simulink library "MotionSimSpatialLibrary"  (Simulink 7.8)
settings: Solver=ode45  StartTime=0.0  StopTime=10.0  RelTol=1e-3
values from neighbouring files (symbols this model uses):
  sysmodel = CalcDof( sysmodel)    [conv2simulink.m]
undefined symbols (not defined in the file or in its folder): selectnum
settings Model: Creator=john  LastModifiedBy=john

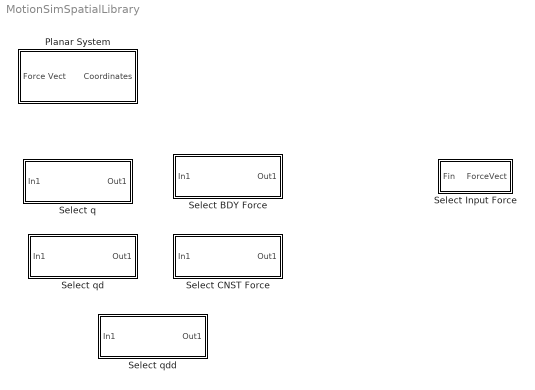
== system MotionSimSpatialLibrary ==
  Planar System : Subsystem
  Select BDY Force : Subsystem  mask{Bodynum=3, Selectnum=Tx}
      mask prompts: Bodynum "Body Number"; Selectnum "Select Coordinate"
      mask StyleString: edit,popup(Fx|Fy|Fz|Tx|Ty|Tz)
      mask Display:
      | port_label('input',1,'Coord');
      | port_label('output',1,'BDY Force');
  Select CNST Force : Subsystem  mask{Bodynum=1, Selectnum=Tx}
      mask prompts: Bodynum "Body Number"; Selectnum "Select Coordinate"
      mask StyleString: edit,popup(Fx|Fy|Fz|Tx|Ty|Tz)
      mask Display:
      | port_label('input',1,'Coord');
      | port_label('output',1,'CNST Force');
  Select Input Force : Subsystem  mask{BodyNum=1, ForceNum=Tx}
      mask prompts: BodyNum "Body Number"; ForceNum "Force"
      mask StyleString: edit,popup(Fx|Fy|Fz|Tx|Ty|Tz)
  Select q : Subsystem  mask{Bodynum=3, Selectnum=X}
      mask prompts: Bodynum "Body Number"; Selectnum "Select Coordinate"
      mask StyleString: edit,popup(X|Y|Z|e0|e1|e2|e3)
      mask Display:
      | port_label('input',1,'Coord');
      | port_label('output',1,'q');
  Select qd : Subsystem  mask{Bodynum=3, Selectnum=Xd}
      mask prompts: Bodynum "Body Number"; Selectnum "Select Coordinate"
      mask StyleString: edit,popup(Xd|Yd|Zd|e0d|e1d|e2d|e3d)
      mask Display:
      | port_label('input',1,'Coord');
      | port_label('output',1,'qd');
  Select qdd : Subsystem  mask{Bodynum=3, Selectnum=Xdd}
      mask prompts: Bodynum "Body Number"; Selectnum "Select Coordinate"
      mask StyleString: edit,popup(Xdd|Ydd|Zdd|e0dd|e1dd|e2dd|e3dd)
      mask Display:
      | port_label('input',1,'Coord');
      | port_label('output',1,'qdd');

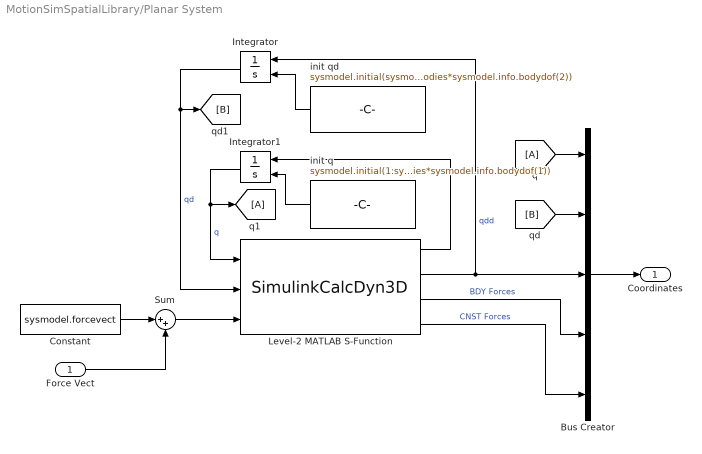
== system MotionSimSpatialLibrary/Planar System ==
  Force Vect : Inport
  Bus Creator : BusCreator  Inputs=5
  Constant : Constant  Value=sysmodel.forcevect
  Integrator : Integrator  InitialConditionSource=external
  Integrator1 : Integrator  InitialConditionSource=external
  Level-2 MATLAB S-Function : M-S-Function  FunctionName=SimulinkCalcDyn3D  Parameters=sysmodel
      mask Display:
      | port_label('output',1,'qd');
      | port_label('output',2,'qdd');
      | port_label('output',3,'Body Forces');
      | port_label('output',4,'Constraint Forces');
      | 
      | port_label('input',1,'q');
      | port_label('input',2,'qd');
  Sum : Sum  Inputs=|++
  init q : Constant  Value=sysmodel.initial(1:sysmodel.info.bodies*sysmodel.info.bodydof(1))
  init qd : Constant  Value=sysmodel.initial(sysmodel.info.bodies*sysmodel.info.bodydof(1)+1:sysmodel.info.bodies*sysmodel.info.bodydof(1)+sysmodel.info.bodies*sysmodel.info.bodydof(2))
  Coordinates : Outport
  wires:
  Bus Creator/1 -> Coordinates/1
  [A] -> Bus Creator/1
  [B] -> Bus Creator/2
  Constant/1 -> Sum/1
  Force Vect/1 -> Sum/2
  Sum/1 -> Level-2 MATLAB S-Function/3
  Level-2 MATLAB S-Function/4 -> Bus Creator/5  "CNST Forces"
  Level-2 MATLAB S-Function/3 -> Bus Creator/4  "BDY Forces"
  init qd/1 -> Integrator/2
  init q/1 -> Integrator1/2
  Level-2 MATLAB S-Function/2 -> Bus Creator/3, Integrator/1  "qdd"
  Level-2 MATLAB S-Function/1 -> Integrator1/1
  Integrator/1 -> [B], Level-2 MATLAB S-Function/2  "qd"
  Integrator1/1 -> [A], Level-2 MATLAB S-Function/1  "q"

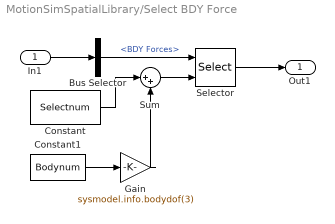
== system MotionSimSpatialLibrary/Select BDY Force ==
  In1 : Inport
  Bus Selector : BusSelector  OutputSignals=BDY Forces
  Constant : Constant  Value=Selectnum
  Constant1 : Constant  Value=Bodynum
  Gain : Gain  Gain=sysmodel.info.bodydof(3)
  Selector : Selector  InputPortWidth=sysmodel.info.bodies*sysmodel.info.bodydof(3)  IndexOptions=Index vector (port)  Indices=[Bodynum+selectnum]  OutputSizes=1
  Sum : Sum  Inputs=|++
  Out1 : Outport
  wires:
  Bus Selector/1 -> Selector/1  "<BDY Forces>"
  In1/1 -> Bus Selector/1
  Gain/1 -> Sum/2
  Constant/1 -> Sum/1
  Sum/1 -> Selector/2
  Constant1/1 -> Gain/1
  Selector/1 -> Out1/1

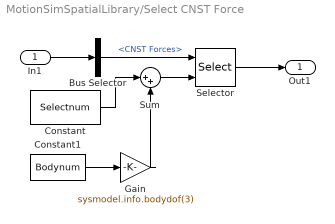
== system MotionSimSpatialLibrary/Select CNST Force ==
  In1 : Inport
  Bus Selector : BusSelector  OutputSignals=CNST Forces
  Constant : Constant  Value=Selectnum
  Constant1 : Constant  Value=Bodynum
  Gain : Gain  Gain=sysmodel.info.bodydof(3)
  Selector : Selector  InputPortWidth=sysmodel.info.bodies*sysmodel.info.bodydof(3)  IndexOptions=Index vector (port)  Indices=[Bodynum+selectnum]  OutputSizes=1
  Sum : Sum  Inputs=|++
  Out1 : Outport
  wires:
  Bus Selector/1 -> Selector/1  "<CNST Forces>"
  In1/1 -> Bus Selector/1
  Gain/1 -> Sum/2
  Constant/1 -> Sum/1
  Sum/1 -> Selector/2
  Constant1/1 -> Gain/1
  Selector/1 -> Out1/1

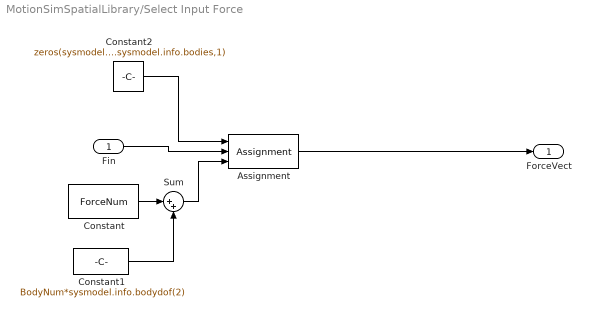
== system MotionSimSpatialLibrary/Select Input Force ==
  Fin : Inport
  Assignment : Assignment  IndexOptions=Index vector (port)  Indices=9  OutputSizes=1
  Constant : Constant  Value=ForceNum
  Constant1 : Constant  Value=BodyNum*sysmodel.info.bodydof(2)
  Constant2 : Constant  Value=zeros(sysmodel.info.bodydof(2)*sysmodel.info.bodies,1)
  Sum : Sum  Inputs=|++
  ForceVect : Outport
  wires:
  Sum/1 -> Assignment/3
  Constant/1 -> Sum/1
  Constant1/1 -> Sum/2
  Fin/1 -> Assignment/2
  Constant2/1 -> Assignment/1
  Assignment/1 -> ForceVect/1

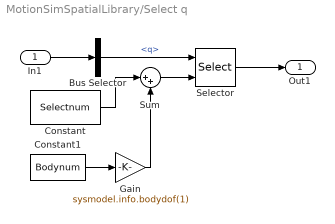
== system MotionSimSpatialLibrary/Select q ==
  In1 : Inport
  Bus Selector : BusSelector  OutputSignals=q
  Constant : Constant  Value=Selectnum
  Constant1 : Constant  Value=Bodynum
  Gain : Gain  Gain=sysmodel.info.bodydof(1)
  Selector : Selector  InputPortWidth=sysmodel.info.bodies*sysmodel.info.bodydof(1)  IndexOptions=Index vector (port)  Indices=[Bodynum+selectnum]  OutputSizes=1
  Sum : Sum  Inputs=|++
  Out1 : Outport
  wires:
  Bus Selector/1 -> Selector/1  "<q>"
  In1/1 -> Bus Selector/1
  Gain/1 -> Sum/2
  Constant/1 -> Sum/1
  Sum/1 -> Selector/2
  Constant1/1 -> Gain/1
  Selector/1 -> Out1/1

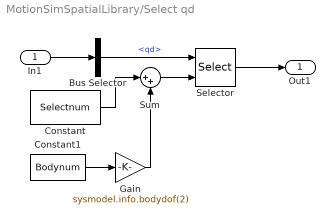
== system MotionSimSpatialLibrary/Select qd ==
  In1 : Inport
  Bus Selector : BusSelector  OutputSignals=qd
  Constant : Constant  Value=Selectnum
  Constant1 : Constant  Value=Bodynum
  Gain : Gain  Gain=sysmodel.info.bodydof(2)
  Selector : Selector  InputPortWidth=sysmodel.info.bodies*sysmodel.info.bodydof(2)  IndexOptions=Index vector (port)  Indices=[Bodynum+selectnum]  OutputSizes=1
  Sum : Sum  Inputs=|++
  Out1 : Outport
  wires:
  Bus Selector/1 -> Selector/1  "<qd>"
  In1/1 -> Bus Selector/1
  Gain/1 -> Sum/2
  Constant/1 -> Sum/1
  Sum/1 -> Selector/2
  Constant1/1 -> Gain/1
  Selector/1 -> Out1/1

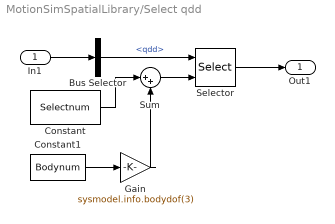
== system MotionSimSpatialLibrary/Select qdd ==
  In1 : Inport
  Bus Selector : BusSelector  OutputSignals=qdd
  Constant : Constant  Value=Selectnum
  Constant1 : Constant  Value=Bodynum
  Gain : Gain  Gain=sysmodel.info.bodydof(3)
  Selector : Selector  InputPortWidth=sysmodel.info.bodies*sysmodel.info.bodydof(3)  IndexOptions=Index vector (port)  Indices=[Bodynum+selectnum]  OutputSizes=1
  Sum : Sum  Inputs=|++
  Out1 : Outport
  wires:
  Bus Selector/1 -> Selector/1  "<qdd>"
  In1/1 -> Bus Selector/1
  Gain/1 -> Sum/2
  Constant/1 -> Sum/1
  Sum/1 -> Selector/2
  Constant1/1 -> Gain/1
  Selector/1 -> Out1/1
